simulink model "ExampleInternalPhysics"  (Simulink 9.2)
settings: Solver=FixedStepDiscrete  StartTime=0.0  StopTime=inf  FixedStep=0.001  RelTol=1e-3  EnableMultiTasking=on
libraries: rFproPhysicsLib x5
settings Model: Creator=enewton  LastModifiedBy=SeanKavanagh
settings OptimizationCC: ExpressionDepthLimit=2147483647  EfficientFloat2IntCast=on
settings DebuggingCC: SolverPrmCheckMsg=warning
settings RTWCC: SystemTargetFile=rfpro.tlc  MakeCommand="make_rtw OPTS=\"-DRUN_PHYSICS\""  TemplateMakefile=rfpro.tmf  Description=rFpro Target (Run Physics)  TargetLang=C++
settings STFCustomTargetCC: ModelReferenceCompliant=off  GeneratePreprocessorConditionals=Disable all  CombineOutputUpdateFcns=on  MatFileLogging=on  CPPClassGenCompliant=on  GRTInterface=off  SystemTargetFile=rfpro.tlc
settings GRTTargetCC: ModelReferenceCompliant=off  ParMdlRefBuildCompliant=off  CompOptLevelCompliant=off  ConcurrentExecutionCompliant=off  CombineOutputUpdateFcns=on  GRTInterface=off  UseToolchainInfoCompliant=off

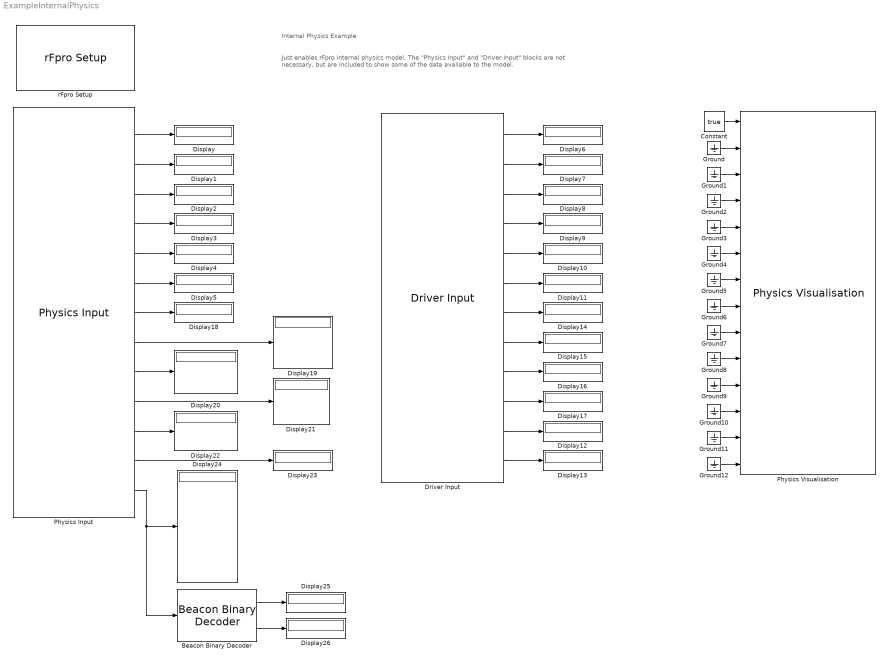
== system ExampleInternalPhysics ==
  note: Internal Physics Example
  note: Just enables rFpro internal physics model.
      | The "Physics Input" and "Driver Input" blocks are not necessary,
      | but are included to show some of the data available to the model.
  Beacon Binary Decoder : rFproPhysicsLib/Beacon Binary Decoder  SystemSampleTime=-1
  Constant : Constant  Value=true
  Display{,1..26} (27 alike) : Display
  Driver Input : rFproPhysicsLib/Driver Input
  Ground{,1..12} (13 alike) : Ground
  Physics Input : rFproPhysicsLib/Physics Input
  Physics Visualisation : rFproPhysicsLib/Physics Visualisation  PAR_SKIP_INTERNAL_PHYSICS=off  PAR_ACCEL_VALID=off  PAR_ROT_ACCEL_VALID=off  PAR_GEAR_VALID=off  PAR_RPM_VALID=off  PAR_INPUTS_VALID=off  PAR_STEER_TORQUE_VALID=off  PAR_HEADLIGHTS_ON_VALID=off  PAR_WHEEL_POS_VALID=off  PAR_WHEEL_ORI_VALID=off  PAR_TYRE_PARAMS_VALID=off  PAR_WHEEL_ROTATION_VALID=off  PAR_WHEEL_BRAKE_TEMP_VALID=off  PAR_WHEEL_TREAD_TEMP_VALID=off  PAR_WHEEL_AIR_TEMP_VALID=off  period=-1  offset=0  useReverseByteOrder=on  rFpro__platform=Remote Model - Default
  rFpro Setup : rFproPhysicsLib/rFpro Setup  platform=Remote Model - Default  stopOnSessionEnd=on  usePseudoRealtime=on  syncToRF=on  useReverseByteOrder=off  useRfTime=on  minIterations=4  maxIterations=1000  ipReceiveAddress='127.0.0.1'  ipReceivePort=11054  receiveSampleTime=-1  ipTransmitAddress='127.0.0.1'  ipTransmitPort=11052  transmitSampleTime=-1  pluginType=RUN_PHYSICS  sysTarget=xpctarget.tlc  templateMakeFile=xpc_default_tmf  makeCommand=make_rtw  buildDesc=xPC target
  wires:
  Constant/1 -> Physics Visualisation/1
  Ground/1 -> Physics Visualisation/2
  Ground1/1 -> Physics Visualisation/3
  Ground2/1 -> Physics Visualisation/4
  Ground3/1 -> Physics Visualisation/5
  Ground4/1 -> Physics Visualisation/6
  Ground5/1 -> Physics Visualisation/7
  Ground6/1 -> Physics Visualisation/8
  Ground7/1 -> Physics Visualisation/9
  Ground8/1 -> Physics Visualisation/10
  Ground9/1 -> Physics Visualisation/11
  Ground10/1 -> Physics Visualisation/12
  Ground11/1 -> Physics Visualisation/13
  Ground12/1 -> Physics Visualisation/14
  Physics Input/1 -> Display/1
  Physics Input/2 -> Display1/1
  Physics Input/3 -> Display2/1
  Physics Input/4 -> Display3/1
  Physics Input/5 -> Display4/1
  Physics Input/6 -> Display5/1
  Driver Input/1 -> Display6/1
  Driver Input/2 -> Display7/1
  Driver Input/3 -> Display8/1
  Driver Input/4 -> Display9/1
  Driver Input/5 -> Display10/1
  Driver Input/6 -> Display11/1
  Driver Input/7 -> Display14/1
  Driver Input/8 -> Display15/1
  Driver Input/9 -> Display16/1
  Driver Input/10 -> Display17/1
  Driver Input/11 -> Display12/1
  Driver Input/12 -> Display13/1
  Physics Input/7 -> Display18/1
  Physics Input/8 -> Display19/1
  Physics Input/9 -> Display20/1
  Physics Input/10 -> Display21/1
  Physics Input/11 -> Display22/1
  Physics Input/12 -> Display23/1
  Physics Input/13 -> Beacon Binary Decoder/1, Display24/1
  Beacon Binary Decoder/1 -> Display25/1
  Beacon Binary Decoder/2 -> Display26/1
